simulink model "SSRobustModelDigital"  (R2020b)
settings: Solver=ode45  StartTime=0.0  StopTime=5  MaxStep=0.0001  RelTol=1e-3
values from neighbouring files (symbols this model uses):
  Ts = T2    (= 0.01)    [PIDAntiWindupDigital.m]    (also in PIDDigital.m = 0.001; StateSpaceControllerNominalCont.m = 0.001; StateSpaceControllerNominalDigital.m = 0.001; StateSpaceControllerNominalDirectDigital.m = 0.05)
settings Model: Creator=umberto  LastModifiedBy=umbe

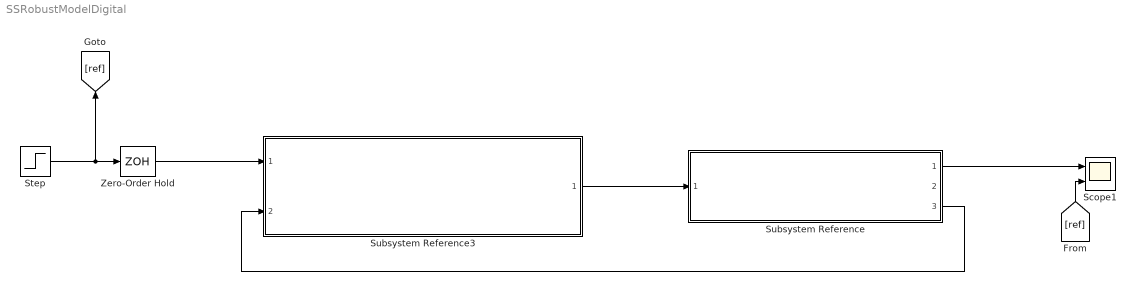
== system SSRobustModelDigital ==
  Scope1 : Scope  NumInputPorts=2
  Step : Step  After=50  SampleTime=0
  Subsystem Reference : Subsystem  ReferencedSubsystem=DCServoMotor_SubSystem
  Subsystem Reference3 : Subsystem  ReferencedSubsystem=RegulatorRobustDigital_SubSystem
  Zero-Order Hold : ZeroOrderHold  SampleTime=Ts
  wires:
  Subsystem Reference3/1 -> Subsystem Reference/1
  Step/1 -> Zero-Order Hold/1, [ref]
  Subsystem Reference/1 -> Scope1/1
  [ref] -> Scope1/2
  Subsystem Reference/3 -> Subsystem Reference3/2
  Zero-Order Hold/1 -> Subsystem Reference3/1
